simulink model "nonlinear_try"  (R2018a)
settings: Solver=VariableStepAuto  StartTime=0.0  StopTime=16.0  RelTol=1e-3
settings Model: Creator=ASUS  LastModifiedBy=ASUS

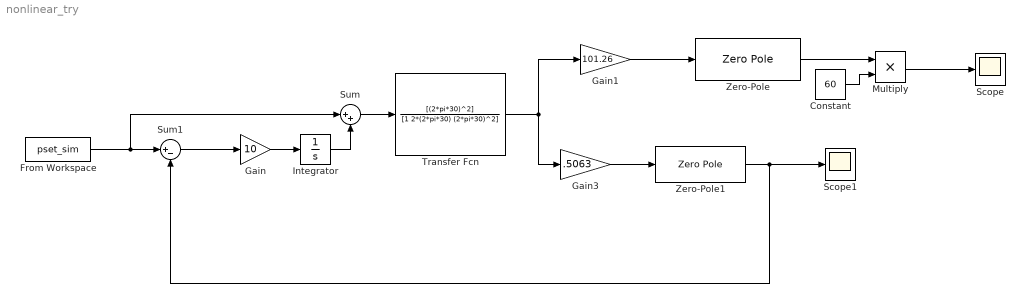
== system nonlinear_try ==
  Constant : Constant  Value=60
  From Workspace : FromWorkspace  VariableName=pset_sim  SampleTime=0
  Gain : Gain  Gain=10
  Gain1 : Gain  Gain=101.26
  Gain3 : Gain  Gain=.5063
  Integrator : Integrator
  Multiply : Product
  Scope : Scope
  Scope1 : Scope
  Sum : Sum  Inputs=|++
  Sum1 : Sum  Inputs=|+-
  Transfer Fcn : TransferFcn  Numerator=[(2*pi*30)^2]  Denominator=[1 2*(2*pi*30) (2*pi*30)^2]
  Zero-Pole : ZeroPole  Zeros=[-8.88e-16]  Poles=[-5.4436]
  Zero-Pole1 : ZeroPole  Zeros=[-10]  Poles=[-5.4436]
  wires:
  Gain/1 -> Integrator/1
  Integrator/1 -> Sum/2
  Sum/1 -> Transfer Fcn/1
  Gain1/1 -> Zero-Pole/1
  Gain3/1 -> Zero-Pole1/1
  Transfer Fcn/1 -> Gain3/1, Gain1/1
  Sum1/1 -> Gain/1
  Zero-Pole1/1 -> Scope1/1, Sum1/2
  From Workspace/1 -> Sum/1, Sum1/1
  Zero-Pole/1 -> Multiply/1
  Constant/1 -> Multiply/2
  Multiply/1 -> Scope/1
